simulink model "Calculator_Model"  (R2021a)
settings: Solver=FixedStepDiscrete  StartTime=0.0  StopTime=10.0  RelTol=1e-3
libraries: simulink x2
settings Model: Creator=Moamen_Hamed  LastModifiedBy=Mahmoud Shams El-Din
settings OptimizationCC: DefaultParameterBehavior=Inlined  EnhancedBackFolding=on  PassReuseOutputArgsAs=Individual arguments  OptimizeBlockOrder=speed  DifferentSizesBufferReuse=on  OptimizationCustomize=off  EfficientTunableParamExpr=on
settings DebuggingCC: ParameterTunabilityLossMsg=error
settings SFSimCC: MATLABDynamicMemAlloc=off
settings RTWCC: SystemTargetFile=ert.tlc  GenCodeOnly=on  TemplateMakefile=ert_default_tmf  GenerateReport=on  IncludeHyperlinkInReport=on  LaunchReport=on  GenerateTraceInfo=on
settings CodeAppCC: ForceParamTrailComments=on  IgnoreCustomStorageClasses=off  OperatorAnnotations=on  SimulinkDataObjDesc=on  SFDataObjDesc=on  InsertBlockDesc=on
settings ERTTargetCC: TargetLangStandard=C99 (ISO)  GenerateSampleERTMain=on  CodeInterfacePackaging=Reusable function  SupportComplex=off  InlinedParameterPlacement=NonHierarchical  ERTCustomFileTemplate=example_file_process.tlc

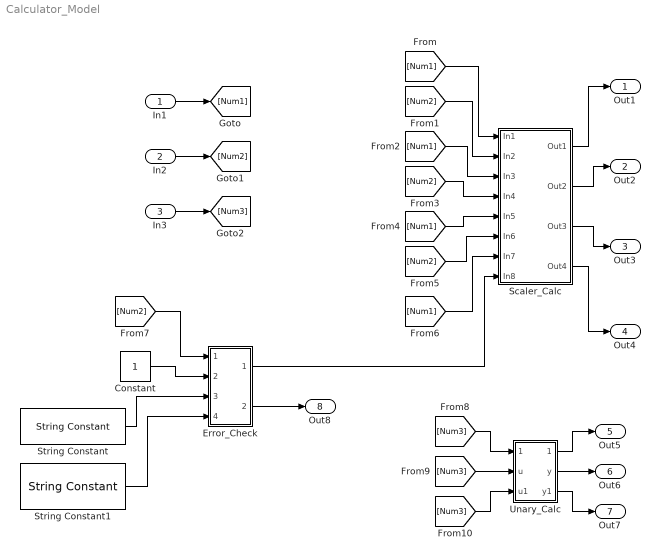
== system Calculator_Model ==
  In1 : Inport  PortDimensions=1
  In2 : Inport  Port=2  PortDimensions=1
  In3 : Inport  Port=3  PortDimensions=1
  Constant : Constant
  Error_Check : Subsystem  TreatAsAtomicUnit=on
  Scaler_Calc : Subsystem  TreatAsAtomicUnit=on
  String Constant : StringConstant  String="\"No Errors!\""
  String Constant1 : StringConstant  String="\"Can't Divide by Zero!\""
  Unary_Calc : Subsystem  TreatAsAtomicUnit=on
  Out1 : Outport  SignalName=Add_Out
  Out2 : Outport  Port=2  SignalName=Sub_Out
  Out3 : Outport  Port=3  SignalName=Prod_Out
  Out4 : Outport  Port=4  SignalName=Div_Out
  Out5 : Outport  Port=5  SignalName=UMinus_Out
  Out6 : Outport  Port=6  SignalName=Incr_Out
  Out7 : Outport  Port=7  SignalName=Decr_Out
  Out8 : Outport  Port=8  SignalName=Error_Out
  wires:
  In1/1 -> [Num1]
  In3/1 -> [Num3]
  In2/1 -> [Num2]
  [Num1] -> Scaler_Calc/1(In1)
  [Num2] -> Scaler_Calc/2(In2)
  [Num1] -> Scaler_Calc/3(In3)
  [Num2] -> Scaler_Calc/4(In4)
  [Num1] -> Scaler_Calc/5(In5)
  [Num2] -> Scaler_Calc/6(In6)
  [Num1] -> Scaler_Calc/7(In7)
  Scaler_Calc/1(Out1) -> Out1/1
  Scaler_Calc/2(Out2) -> Out2/1
  Scaler_Calc/3(Out3) -> Out3/1
  Scaler_Calc/4(Out4) -> Out4/1
  [Num3] -> Unary_Calc/1(In1)
  [Num3] -> Unary_Calc/2(u)
  [Num3] -> Unary_Calc/3(u1)
  Unary_Calc/1(Out1) -> Out5/1
  Unary_Calc/2(y) -> Out6/1
  Unary_Calc/3(y1) -> Out7/1
  [Num2] -> Error_Check/1(In1)
  Constant/1 -> Error_Check/2(In2)
  String Constant/1 -> Error_Check/3(In3)
  String Constant1/1 -> Error_Check/4(In4)
  Error_Check/1(Out1) -> Scaler_Calc/8(In8)
  Error_Check/2(Out2) -> Out8/1

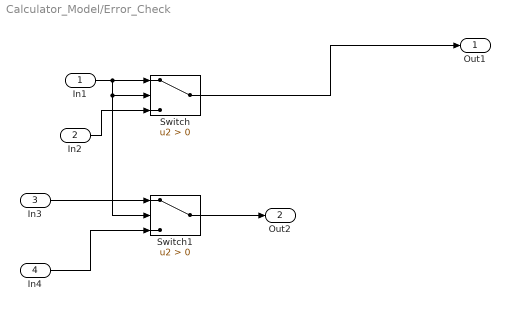
== system Calculator_Model/Error_Check ==
  In1 : Inport
  In2 : Inport  Port=2
  In3 : Inport  Port=3
  In4 : Inport  Port=4
  Switch : Switch  Criteria=u2 > Threshold
  Switch1 : Switch  Criteria=u2 > Threshold
  Out1 : Outport
  Out2 : Outport  Port=2
  wires:
  Switch/1 -> Out1/1
  In3/1 -> Switch1/1
  In1/1 -> Switch1/2, Switch/2, Switch/1
  Switch1/1 -> Out2/1
  In2/1 -> Switch/3
  In4/1 -> Switch1/3

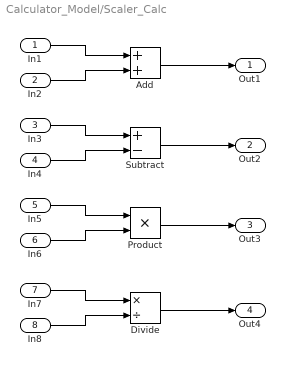
== system Calculator_Model/Scaler_Calc ==
  In1 : Inport
  In2 : Inport  Port=2
  In3 : Inport  Port=3
  In4 : Inport  Port=4
  In5 : Inport  Port=5
  In6 : Inport  Port=6
  In7 : Inport  Port=7
  In8 : Inport  Port=8
  Add : Sum
  Divide : Product  Inputs=*/
  Product : Product
  Subtract : Sum  Inputs=+-
  Out1 : Outport
  Out2 : Outport  Port=2
  Out3 : Outport  Port=3
  Out4 : Outport  Port=4
  wires:
  Divide/1 -> Out4/1
  In8/1 -> Divide/2
  In7/1 -> Divide/1
  Add/1 -> Out1/1
  In3/1 -> Subtract/1
  In1/1 -> Add/1
  Product/1 -> Out3/1
  In4/1 -> Subtract/2
  In5/1 -> Product/1
  Subtract/1 -> Out2/1
  In2/1 -> Add/2
  In6/1 -> Product/2

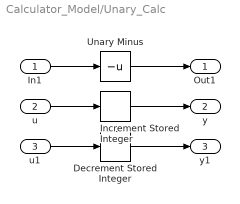
== system Calculator_Model/Unary_Calc ==
  In1 : Inport
  u : Inport  Port=2
  u1 : Inport  Port=3
  Decrement Stored Integer : simulink/Additional Math & Discrete/Additional Math: Increment - Decrement/Decrement Stored Integer
      settings: SourceProductBaseCode=SL
  Increment Stored Integer : simulink/Additional Math & Discrete/Additional Math: Increment - Decrement/Increment Stored Integer
  Unary Minus : UnaryMinus
  Out1 : Outport
  y : Outport  Port=2
  y1 : Outport  Port=3
  wires:
  In1/1 -> Unary Minus/1
  Unary Minus/1 -> Out1/1
  Increment Stored Integer/1 -> y/1
  Decrement Stored Integer/1 -> y1/1
  u1/1 -> Decrement Stored Integer/1
  u/1 -> Increment Stored Integer/1
